simulink model "task1"  (R2019b)
settings: Solver=VariableStepAuto  StartTime=0.0  StopTime=18*100  RelTol=1e-3
undefined symbols (not defined in the file): DiscIntNeverNeededParam
libraries: simulink x9, dspswit3 x1, commrandsrc3 x1
settings Model: Creator=ZB  LastModifiedBy=ZB

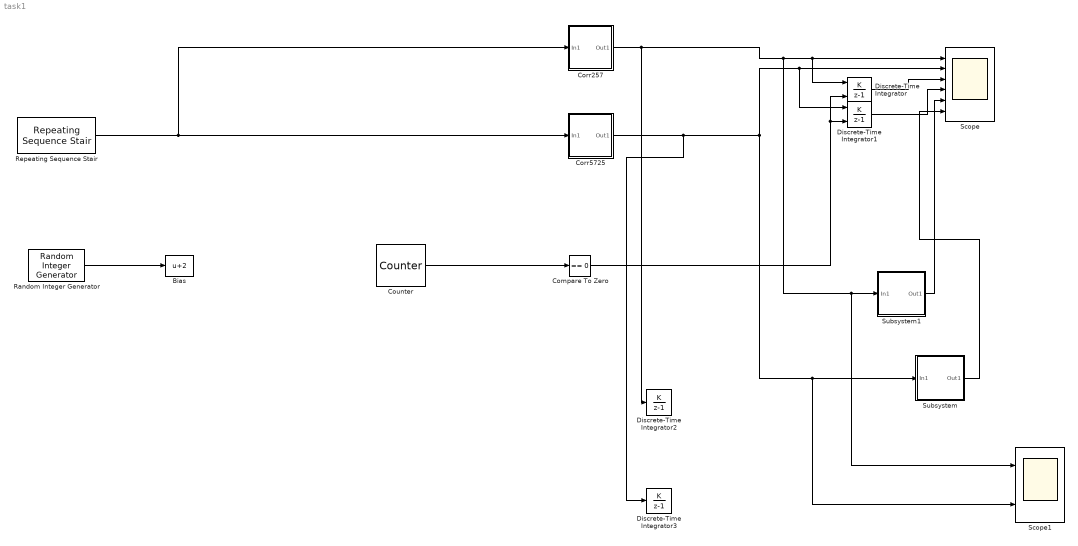
== system task1 ==
  Bias : Bias  Bias=2
  Compare To Zero : simulink/Logic and Bit Operations/Compare To Zero  relop===  OutDataTypeStr=boolean
  Corr257 : Subsystem
  Corr5725 : Subsystem
  Counter : dspswit3/Counter  Direction=Up  CountEvent=Free running  CounterSize=User defined  MaxCount=17  InitialCount=0  Output=Count  HitValue=32  ResetInput=off  SamplesPerFrame=1  Ts=1  CntDtype=double  HitDtype=Logical
  Discrete-Time Integrator : DiscreteIntegrator  IntegratorMethod=Accumulation: Forward Euler  ExternalReset=rising  SampleTime=-1  ICPrevOutput=DiscIntNeverNeededParam  ICPrevScaledInput=DiscIntNeverNeededParam
  Discrete-Time Integrator1 : DiscreteIntegrator  IntegratorMethod=Accumulation: Forward Euler  ExternalReset=rising  SampleTime=-1  ICPrevOutput=DiscIntNeverNeededParam  ICPrevScaledInput=DiscIntNeverNeededParam
  Discrete-Time Integrator2 : DiscreteIntegrator  IntegratorMethod=Accumulation: Forward Euler  SampleTime=-1  ICPrevOutput=DiscIntNeverNeededParam  ICPrevScaledInput=DiscIntNeverNeededParam
  Discrete-Time Integrator3 : DiscreteIntegrator  IntegratorMethod=Accumulation: Forward Euler  SampleTime=-1  ICPrevOutput=DiscIntNeverNeededParam  ICPrevScaledInput=DiscIntNeverNeededParam
  Random Integer Generator : commrandsrc3/Random Integer Generator  SetSize=6  SeedSource=Auto  Seed=0  SampleTime=1  SamplesPerFrame=1  OutputDataType=double  SimulateUsing=Interpreted execution
      settings: SourceProductName=Communications Toolbox
  Repeating Sequence Stair : simulink/Sources/Repeating Sequence Stair  OutValues=[2 5 7 2 5 3 8 7 2 5 7 2 3 5 7 2 5 7]'  tsamp=1  OutMin=[]  OutMax=[]  OutDataTypeStr=double  OutputDataTypeScalingMode=double  OutDataType=fixdt(0,8)  ConRadixGroup=Best Precision: Vector-wise  OutScaling=2^-12
  Scope : Scope  NumInputPorts=6
  Scope1 : Scope  NumInputPorts=2
  Subsystem : Subsystem  mask{a=0.01}
  Subsystem1 : Subsystem  mask{a=0.01}
  wires:
  Random Integer Generator/1 -> Bias/1
  Corr257/1(Out1) -> Discrete-Time Integrator2/1, Scope1/1, Subsystem1/1(In1), Scope/1, Discrete-Time Integrator/1
  Corr5725/1(Out1) -> Discrete-Time Integrator3/1, Scope1/2, Subsystem/1(In1), Scope/2, Discrete-Time Integrator1/1
  Discrete-Time Integrator/1 -> Scope/3
  Discrete-Time Integrator1/1 -> Scope/4
  Counter/1 -> Compare To Zero/1
  Compare To Zero/1 -> Discrete-Time Integrator1/2, Discrete-Time Integrator/2
  Subsystem/1(Out1) -> Scope/6
  Subsystem1/1(Out1) -> Scope/5
  Repeating Sequence Stair/1 -> Corr5725/1(In1), Corr257/1(In1)

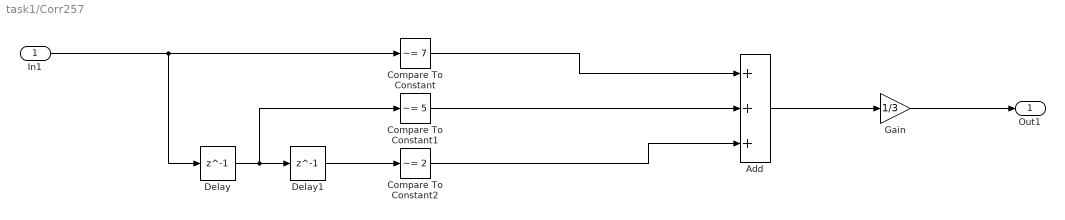
== system task1/Corr257 ==
  In1 : Inport
  Add : Sum  Inputs=+++  AccumDataTypeStr=double  OutDataTypeStr=Inherit: Same as accumulator
  Compare To Constant : simulink/Logic and Bit Operations/Compare To Constant  relop=~=  const=7  OutDataTypeStr=boolean
  Compare To Constant1 : simulink/Logic and Bit Operations/Compare To Constant  relop=~=  const=5  OutDataTypeStr=boolean
  Compare To Constant2 : simulink/Logic and Bit Operations/Compare To Constant  relop=~=  const=2  OutDataTypeStr=boolean
  Delay : Delay  DelayLength=1  InitialCondition=0
  Delay1 : Delay  DelayLength=1  InitialCondition=0
  Gain : Gain  Gain=1/3
  Out1 : Outport
  wires:
  Delay/1 -> Compare To Constant1/1, Delay1/1
  In1/1 -> Delay/1, Compare To Constant/1
  Delay1/1 -> Compare To Constant2/1
  Add/1 -> Gain/1
  Compare To Constant/1 -> Add/1
  Compare To Constant1/1 -> Add/2
  Compare To Constant2/1 -> Add/3
  Gain/1 -> Out1/1

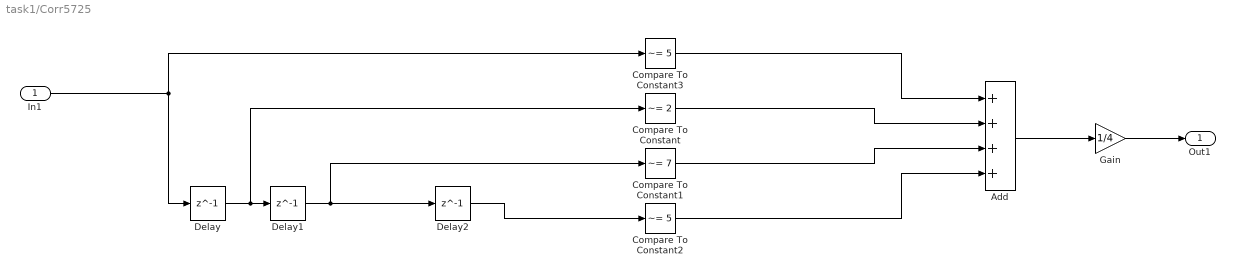
== system task1/Corr5725 ==
  In1 : Inport
  Add : Sum  Inputs=++++  AccumDataTypeStr=double  OutDataTypeStr=Inherit: Same as accumulator
  Compare To Constant : simulink/Logic and Bit Operations/Compare To Constant  relop=~=  const=2  OutDataTypeStr=boolean
  Compare To Constant1 : simulink/Logic and Bit Operations/Compare To Constant  relop=~=  const=7  OutDataTypeStr=boolean
  Compare To Constant2 : simulink/Logic and Bit Operations/Compare To Constant  relop=~=  const=5  OutDataTypeStr=boolean
  Compare To Constant3 : simulink/Logic and Bit Operations/Compare To Constant  relop=~=  const=5  OutDataTypeStr=boolean
  Delay : Delay  DelayLength=1  InitialCondition=0
  Delay1 : Delay  DelayLength=1  InitialCondition=0
  Delay2 : Delay  DelayLength=1  InitialCondition=0
  Gain : Gain  Gain=1/4
  Out1 : Outport
  wires:
  Compare To Constant2/1 -> Add/4
  Compare To Constant1/1 -> Add/3
  Compare To Constant/1 -> Add/2
  Add/1 -> Gain/1
  Delay1/1 -> Delay2/1, Compare To Constant1/1
  In1/1 -> Compare To Constant3/1, Delay/1
  Delay/1 -> Delay1/1, Compare To Constant/1
  Compare To Constant3/1 -> Add/1
  Delay2/1 -> Compare To Constant2/1
  Gain/1 -> Out1/1

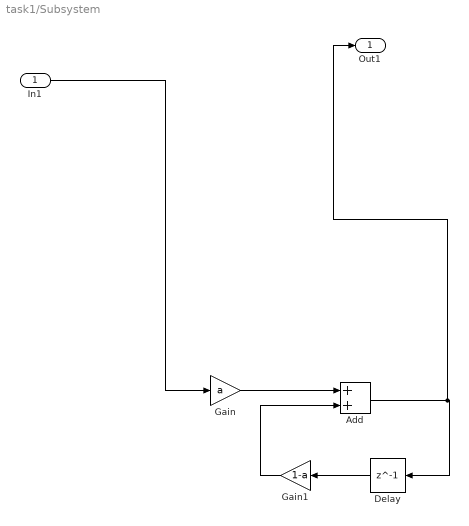
== system task1/Subsystem ==
  In1 : Inport
  Add : Sum
  Delay : Delay  DelayLength=1
  Gain : Gain  Gain=a
  Gain1 : Gain  Gain=1-a
  Out1 : Outport
  wires:
  Add/1 -> Out1/1, Delay/1
  Gain1/1 -> Add/2
  In1/1 -> Gain/1
  Delay/1 -> Gain1/1
  Gain/1 -> Add/1

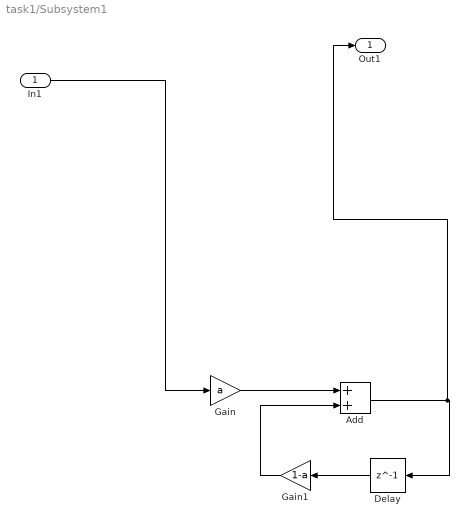
== system task1/Subsystem1 ==
  In1 : Inport
  Add : Sum
  Delay : Delay  DelayLength=1
  Gain : Gain  Gain=a
  Gain1 : Gain  Gain=1-a
  Out1 : Outport
  wires:
  Gain/1 -> Add/1
  Delay/1 -> Gain1/1
  In1/1 -> Gain/1
  Gain1/1 -> Add/2
  Add/1 -> Delay/1, Out1/1
